simulink model "OneWheelTCSMT"  (R2022b)
settings: Solver=ode45  StartTime=0.0  StopTime=5  MaxStep=.01  RelTol=1e-3  AbsTol=1e-6
PreLoadFcn:
  | load('OneWheelTCS.mat')
undefined symbols (not defined in the file): B, C, ctrl, D, E, I, Kf, m, PBmax, Rr, Sh, Sv, TB, v0, w0
libraries: slpidlib x1
settings Model: Creator=ctrapeni  LastModifiedBy=brianlesko
settings SolverCC: AlgebraicLoopSolver=TrustRegion
settings DataIOCC: SaveFormat=Array  SignalLoggingSaveFormat=ModelDataLogs  SaveOutput=off  ReturnWorkspaceOutputs=off  TimeSaveName=time  SignalLoggingName=sigsOut
settings DebuggingCC: SaveWithParameterizedLinksMsg=none  UnderspecifiedInitializationDetection=Classic  MergeDetectMultiDrivingBlocksExec=none  SignalResolutionControl=TryResolveAllWithWarning  MultiTaskDSMMsg=warning  MultiTaskCondExecSysMsg=none  IntegerOverflowMsg=none  UnconnectedInputMsg=warning  UnconnectedOutputMsg=warning  UnconnectedLineMsg=warning  SFMachineParentedDataDiag=warning
settings HardwareCC: ProdBitPerPointer=32  ProdBitPerSizeT=32  ProdBitPerPtrDiffT=32  ProdLargestAtomicFloat=None  ProdIntDivRoundTo=Undefined  ProdEndianess=Unspecified  ProdWordSize=32  ProdHWDeviceType=32-bit Generic  TargetUnknown=on
settings ModelReferenceCC: EnableRefExpFcnMdlSchedulingChecks=on  PropagateSignalLabelsOutOfModel=off
settings RTWCC: DLArmComputeVersion=19.05
settings GRTTargetCC: CombineOutputUpdateFcns=off  GRTInterface=on
settings ConfigComp: CovMetricSettings=dw  CovSaveCumulativeToWorkspaceVar=on  CovSaveSingleToWorkspaceVar=on

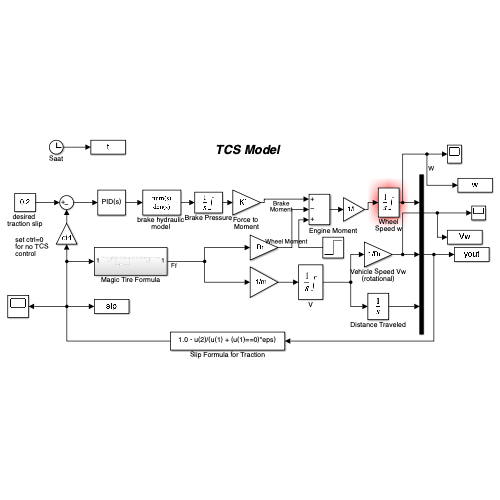
[thumbnail: Simulink's stored preview of the top-level diagram]
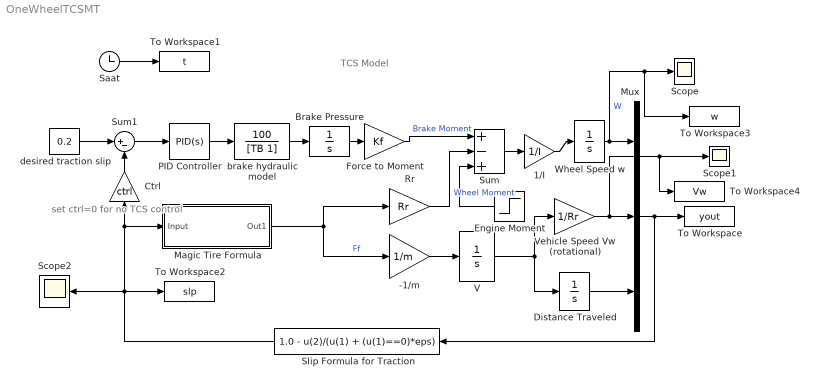
== system OneWheelTCSMT ==
  note: TCS Model
  note: set ctrl=0
      | for no TCS
      | control
  -1/m : Gain  Gain=1/m  SaturateOnIntegerOverflow=on  OutDataTypeStr=Inherit: Same as input  ParamDataTypeStr=Inherit: Same as input
  1/I : Gain  Gain=1/I  SaturateOnIntegerOverflow=on  OutDataTypeStr=Inherit: Same as input  ParamDataTypeStr=Inherit: Same as input
  Brake Pressure : Integrator  LimitOutput=on  UpperSaturationLimit=0  LowerSaturationLimit=-PBmax
  Ctrl : Gain  Gain=ctrl  SaturateOnIntegerOverflow=on  OutDataTypeStr=Inherit: Same as input  ParamDataTypeStr=Inherit: Same as input
  Distance Traveled : Integrator  UpperSaturationLimit=1000  LowerSaturationLimit=0
  Engine Moment : Step  Time=0  After=1000  SampleTime=0
  Force to Moment : Gain  Gain=Kf  SaturateOnIntegerOverflow=on  OutDataTypeStr=Inherit: Same as input  ParamDataTypeStr=Inherit: Same as input
  Magic Tire Formula : Subsystem
  Mux : Mux  Inputs=3
  PID Controller : slpidlib/PID Controller  Controller=PID  Form=Parallel  TimeDomain=Continuous-time  UseExternalTs=off  SampleTime=-1  IntegratorMethod=Forward Euler  FilterMethod=Forward Euler  ControllerParametersSource=internal  P=250  I=1  UseKiTs=off  D=60  N=1000  UseFilter=on  TunerSelectOption=Transfer Function Based (PID Tuner App)  InitialConditionSource=internal  InitialConditionForIntegrator=0  InitialConditionForFilter=0  DifferentiatorICPrevScaledInput=0  ExternalReset=none  TrackingMode=off  Kt=1  LimitOutput=off  SatLimitsSource=internal  UpperSaturationLimit=inf  LowerSaturationLimit=-inf  LinearizeAsGain=on  AntiWindupMode=none  Kb=1  LimitIntegrator=off  UpperIntegratorSaturationLimit=inf  LowerIntegratorSaturationLimit=-inf  POutMin=[]  POutMax=[]  IOutMin=[]  IOutMax=[]  DOutMin=[]  DOutMax=[]  NOutMin=[]  NOutMax=[]  SumOutMin=[]  SumOutMax=[]  SaturationOutMin=[]  SaturationOutMax=[]  PParamMin=[]  PParamMax=[]  IParamMin=[]  IParamMax=[]  DParamMin=[]  DParamMax=[]  NParamMin=[]  NParamMax=[]  KbParamMin=[]  KbParamMax=[]  KtParamMin=[]  KtParamMax=[]  KbOutMin=[]  KbOutMax=[]  KtOutMin=[]  KtOutMax=[]  IntegratorOutMin=[]  IntegratorOutMax=[]  FilterOutMin=[]  FilterOutMax=[]  SumI1OutMin=[]  SumI1OutMax=[]  SumI2OutMin=[]  SumI2OutMax=[]  SumI3OutMin=[]  SumI3OutMax=[]  SumI4OutMin=[]  SumI4OutMax=[]  SumDOutMin=[]  SumDOutMax=[]  DifferentiatorOutMin=[]  DifferentiatorOutMax=[]  FilterDiffOutCoefMin=[]  FilterDiffOutCoefMax=[]  ReciprocalOutMin=[]  ReciprocalOutMax=[]  SumDenOutMin=[]  SumDenOutMax=[]  SumNumOutMin=[]  SumNumOutMax=[]  DivideOutMin=[]  DivideOutMax=[]  UdiffTsProdOutMin=[]  UdiffTsProdOutMax=[]  NTsProdOutMin=[]  NTsProdOutMax=[]  UintegralTsProdOutMin=[]  UintegralTsProdOutMax=[]  UngainTsProdOutMin=[]  UngainTsProdOutMax=[]  ClampingZeroOutDataTypeStr=Inherit: Inherit via back propagation  ClampingZeroOutMin=[]  ClampingZeroOutMax=[]  FilterDenConstantOutDataTypeStr=Inherit: Inherit via back propagation  FilterDenConstantOutMin=[]  FilterDenConstantOutMax=[]  PCopyOutDataTypeStr=Inherit: Inherit via back propagation  PCopyOutMin=[]  PCopyOutMax=[]  NCopyOutDataTypeStr=Inherit: Inherit via back propagation  NCopyOutMin=[]  NCopyOutMax=[]  IntegratorContinuousStateAttributes=''  IntegratorStateMustResolveToSignalObject=off  IntegratorRTWStateStorageClass=Auto  FilterContinuousStateAttributes=''  FilterStateMustResolveToSignalObject=off  FilterRTWStateStorageClass=Auto  ParallelPVariant=InternalParameters  IdealPVariant=Disabled  IVariant=InternalParameters  DVariant=InternalParameters  IntegratorVariant=Continuous  SatVariant=Disabled  AWVariant=Passthrough  PCopyVariant=Disabled  TRVariant=Disabled  FdbkBlocksVariant=Forward  IdealPFdbkVariant=Disabled  SatFdbkVariant=Disabled  DerivativeFilterVariant=ContFilter  NVariant=InternalParameters  NCopyVariant=Disabled  FilterICVariant=InternalICsFilter  IntegratorICVariant=InternalICs  ExternalResetVariant=Disabled  TRSumVariant=Passthrough  SumFdbkVariant=Disabled  SumVariant=Sum_PID  TsampFilterVariant=InternalTs  TsampNgainVariant=Passthrough  TsampIntegralVariant=Passthrough  ExternalSaturationOutDataTypeStr=Inherit: Same as second input
  Rr : Gain  Gain=Rr  SaturateOnIntegerOverflow=on  OutDataTypeStr=Inherit: Same as input  ParamDataTypeStr=Inherit: Same as input
  Saat : Clock
  Scope : Scope
  Scope1 : Scope
  Scope2 : Scope
  Slip Formula for Traction : Fcn  Expr=1.0 - u(2)/(u(1) + (u(1)==0)*eps)
  Sum : Sum  Inputs=+-+  InputSameDT=on  SaturateOnIntegerOverflow=on  OutDataTypeStr=Inherit: Same as first input
  Sum1 : Sum  Inputs=|+-  InputSameDT=on  SaturateOnIntegerOverflow=on  OutDataTypeStr=Inherit: Same as first input
  To Workspace : ToWorkspace  VariableName=yout
      settings: MaxDataPoints=10000
  To Workspace1 : ToWorkspace  VariableName=t
      settings: MaxDataPoints=10000
  To Workspace2 : ToWorkspace  VariableName=slp
      settings: MaxDataPoints=10000
  To Workspace3 : ToWorkspace  VariableName=w
      settings: MaxDataPoints=10000
  To Workspace4 : ToWorkspace  VariableName=Vw
      settings: MaxDataPoints=10000
  V : Integrator  InitialCondition=v0  LimitOutput=on  UpperSaturationLimit=1000  LowerSaturationLimit=0
  Vehicle Speed Vw (rotational) : Gain  Gain=1/Rr  SaturateOnIntegerOverflow=on  OutDataTypeStr=Inherit: Same as input  ParamDataTypeStr=Inherit: Same as input
  Wheel Speed w : Integrator  InitialCondition=w0  LimitOutput=on  UpperSaturationLimit=1000  LowerSaturationLimit=0
  "brake hydraulic model " : TransferFcn  Numerator=[100]  Denominator=[TB 1]
  desired traction slip : Constant  Value=0.2
  wires:
  Saat/1 -> To Workspace1/1
  V/1 -> Vehicle Speed Vw (rotational)/1, Distance Traveled/1
  Rr/1 -> Sum/2  "Wheel Moment"
  PID Controller/1 -> "brake hydraulic model "/1
  desired traction slip/1 -> Sum1/1
  Magic Tire Formula/1(Out1) -> -1/m/1, Rr/1  "Ff"
  Ctrl/1 -> Sum1/2
  Slip Formula for Traction/1 -> Scope2/1, Magic Tire Formula/1(Input), Ctrl/1, To Workspace2/1
  1/I/1 -> Wheel Speed w/1
  Brake Pressure/1 -> Force to Moment/1
  Mux/1 -> To Workspace/1, Slip Formula for Traction/1
  Distance Traveled/1 -> Mux/3
  Wheel Speed w/1 -> Mux/1, Scope/1, To Workspace3/1  "W"
  Force to Moment/1 -> Sum/1  "Brake Moment"
  Vehicle Speed Vw (rotational)/1 -> Mux/2, Scope1/1, To Workspace4/1
  Sum1/1 -> PID Controller/1
  Engine Moment/1 -> Sum/3
  -1/m/1 -> V/1
  "brake hydraulic model "/1 -> Brake Pressure/1
  Sum/1 -> 1/I/1

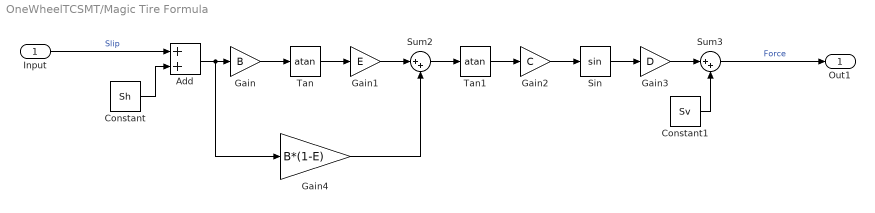
== system OneWheelTCSMT/Magic Tire Formula ==
  Input : Inport
  Add : Sum
  Constant : Constant  Value=Sh
  Constant1 : Constant  Value=Sv
  Gain : Gain  Gain=B
  Gain1 : Gain  Gain=E
  Gain2 : Gain  Gain=C
  Gain3 : Gain  Gain=D
  Gain4 : Gain  Gain=B*(1-E)
  Sin : Trigonometry
  Sum2 : Sum  Inputs=|++
  Sum3 : Sum  Inputs=|++
  Tan : Trigonometry  Operator=atan
  Tan1 : Trigonometry  Operator=atan
  Out1 : Outport
  wires:
  Tan/1 -> Gain1/1
  Sum2/1 -> Tan1/1
  Sum3/1 -> Out1/1  "Force"
  Gain2/1 -> Sin/1
  Gain4/1 -> Sum2/2
  Tan1/1 -> Gain2/1
  Gain1/1 -> Sum2/1
  Constant/1 -> Add/2
  Gain/1 -> Tan/1
  Gain3/1 -> Sum3/1
  Constant1/1 -> Sum3/2
  Add/1 -> Gain4/1, Gain/1
  Sin/1 -> Gain3/1
  Input/1 -> Add/1  "Slip"
